simulink model "second_task"  (R2023a)
settings: Solver=VariableStepAuto  StartTime=0.0  StopTime=Tdes  RelTol=1e-3
undefined symbols (not defined in the file): axang2rotm, j, k1e1, k1e2, k2e1, k2e2, kr, ks, kw, n, nd, q0, vs_des
settings Model: Creator=Nabil Samaan  LastModifiedBy=dvogureckiy99
settings DebuggingCC: UnconnectedInputMsg=warning  UnconnectedOutputMsg=warning  UnconnectedLineMsg=warning
settings ModelReferenceCC: EnableRefExpFcnMdlSchedulingChecks=on
settings RTWCC: DLArmComputeVersion=19.05

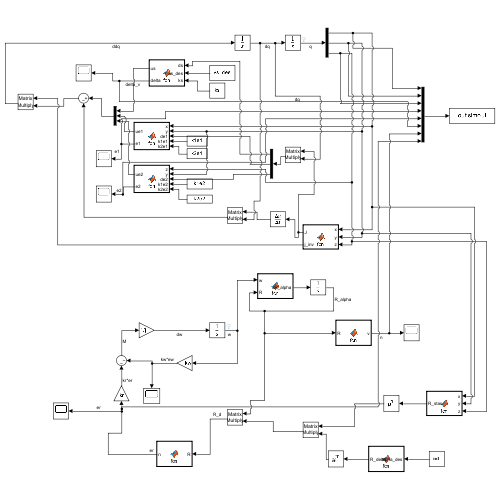
[thumbnail: Simulink's stored preview of the top-level diagram]
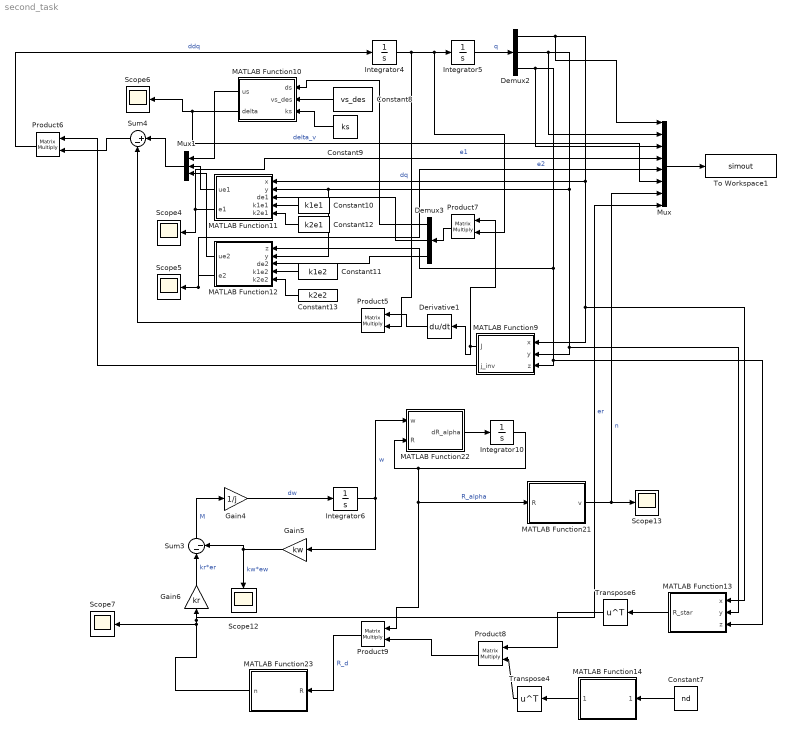
== system second_task ==
  Constant10 : Constant  Value=k1e1
  Constant11 : Constant  Value=k1e2
  Constant12 : Constant  Value=k2e1
  Constant13 : Constant  Value=k2e2
  Constant7 : Constant  Value=nd
  Constant8 : Constant  Value=vs_des
  Constant9 : Constant  Value=ks
  Demux2 : Demux  Outputs=3
  Demux3 : Demux  Outputs=3
  Derivative1 : Derivative  CoefficientInTFapproximation=0.001
  Gain4 : Gain  Gain=1/j
  Gain5 : Gain  Gain=kw
  Gain6 : Gain  Gain=kr
  Integrator10 : Integrator  InitialCondition=axang2rotm([n / norm(n) , norm(n)]);
  Integrator4 : Integrator
  Integrator5 : Integrator  InitialCondition=q0
  Integrator6 : Integrator  InitialCondition=[0;0;0]
  MATLAB Function10 : MATLAB Function  TreatAsAtomicUnit=on
  MATLAB Function11 : MATLAB Function  TreatAsAtomicUnit=on
  MATLAB Function12 : MATLAB Function  TreatAsAtomicUnit=on
  MATLAB Function13 : MATLAB Function  TreatAsAtomicUnit=on
  MATLAB Function14 : MATLAB Function  TreatAsAtomicUnit=on
  MATLAB Function21 : MATLAB Function  TreatAsAtomicUnit=on
  MATLAB Function22 : MATLAB Function  TreatAsAtomicUnit=on
  MATLAB Function23 : MATLAB Function  TreatAsAtomicUnit=on
  MATLAB Function9 : MATLAB Function  TreatAsAtomicUnit=on
  Mux : Mux  Inputs=8
  Mux1 : Mux  Inputs=3
  Product{5..9} (5 alike) : Product  Multiplication=Matrix(*)
  Scope{4..7,12..13} (6 alike) : Scope
  Sum3 : Sum  Inputs=|--
  Sum4 : Sum  Inputs=|+-
  To Workspace1 : ToWorkspace  VariableName=simout  SampleTime=-1
      settings: Save2DSignal=2-D array (concatenate along first dimension)
  Transpose4 : Math  Operator=transpose
  Transpose6 : Math  Operator=transpose
  wires:
  Demux3/1 -> MATLAB Function10/1(ds)
  Constant10/1 -> MATLAB Function11/4(k1e1)
  Gain6/1 -> Sum3/1  "kr*er"
  Product7/1 -> Demux3/1
  MATLAB Function12/2(e2) -> Mux/5, Scope5/1  "e2"
  MATLAB Function14/1(R_delta) -> Transpose4/1
  Gain4/1 -> Integrator6/1  "dw"
  Integrator6/1 -> MATLAB Function22/1(w), Gain5/1  "w"
  Sum3/1 -> Gain4/1  "M"
  MATLAB Function10/2(delta) -> Mux/6, Scope6/1  "delta_v"
  Constant12/1 -> MATLAB Function11/5(k2e1)
  MATLAB Function11/2(e1) -> Scope4/1, Mux/4  "e1"
  Constant13/1 -> MATLAB Function12/5(k2e2)
  MATLAB Function11/1(ue1) -> Mux1/2
  Constant11/1 -> MATLAB Function12/4(k1e2)
  Constant7/1 -> MATLAB Function14/1(alpha_des)
  Gain5/1 -> Scope12/1, Sum3/2  "kw*ew"
  Product6/1 -> Integrator4/1  "ddq"
  Constant9/1 -> MATLAB Function10/3(ks)
  MATLAB Function12/1(ue2) -> Mux1/3
  MATLAB Function9/2(j_inv) -> Product6/1
  Constant8/1 -> MATLAB Function10/2(vs_des)
  Mux1/1 -> Sum4/1
  Demux3/2 -> MATLAB Function11/3(de1)
  Product9/1 -> MATLAB Function23/1(R)  "R_d"
  Derivative1/1 -> Product5/1
  Demux3/3 -> MATLAB Function12/3(de2)
  Product5/1 -> Sum4/2
  MATLAB Function10/1(us) -> Mux1/1
  MATLAB Function9/1(J) -> Derivative1/1, Product7/1
  Integrator5/1 -> Demux2/1  "q"
  Sum4/1 -> Product6/2
  Integrator4/1 -> Product5/2, Product7/2, Integrator5/1  "dq"
  Integrator10/1 -> MATLAB Function22/2(R), MATLAB Function21/1(R), Product9/1  "R_alpha"
  MATLAB Function22/1(dR_alpha) -> Integrator10/1
  MATLAB Function21/1(v) -> Mux/7, Scope13/1  "n"
  Demux2/1 -> Mux/1, MATLAB Function11/1(x), MATLAB Function13/1(x), MATLAB Function9/1(x)
  Demux2/2 -> Mux/2, MATLAB Function9/2(y), MATLAB Function13/2(y), MATLAB Function12/2(y), MATLAB Function11/2(y)
  Demux2/3 -> Mux/3, MATLAB Function12/1(z), MATLAB Function13/3(z), MATLAB Function9/3(z)
  Transpose4/1 -> Product8/2
  MATLAB Function13/1(R_star) -> Transpose6/1
  Transpose6/1 -> Product8/1
  MATLAB Function23/1(n) -> Mux/8, Gain6/1, Scope7/1  "er"
  Product8/1 -> Product9/2
  Mux/1 -> To Workspace1/1

== matlab function second_task/MATLAB Function10 ==
  data: ds input; us output; vs_des input; ks input; delta output
function [us,delta] = fcn(ds,vs_des,ks)

delta=vs_des-ds;

us=ks*delta;

== matlab function second_task/MATLAB Function11 ==
  data: x input; ue1 output; y input; de1 input; k1e1 input; k2e1 input; e1 output
function [ue1,e1] = fcn(x,y,de1,k1e1,k2e1)

e1= 0.4*x^2 + 0.8*y^2 -225;
ue1=-k1e1*de1-k2e1*e1;

== matlab function second_task/MATLAB Function12 ==
  data: z input; ue2 output; y input; de2 input; k1e2 input; k2e2 input; e2 output
function [ue2,e2] = fcn(z,y,de2,k1e2,k2e2)

e2= z+0.25*y^2-3;
ue2=-k1e2*de2-k2e2*e2;

== matlab function second_task/MATLAB Function13 ==
  data: x input; R_star output; y input; z input
function R_star= fcn(x,y,z)

gf1=[0.8*x;1.6*y;0];
gf2=[0;0.5*y;1];
c=cross(gf1,gf2);
j1=c/norm(c);
j2=gf1/norm(gf1);
cc=cross(c,gf1);
j3=cc/norm(cc);

R_star=[j1';j2';j3'];

== matlab function second_task/MATLAB Function14 ==
  data: alpha_des input; R_delta output
function R_delta = fcn(alpha_des)


R_delta= axang2rotm([alpha_des' / norm(alpha_des) , norm(alpha_des)]);

== matlab function second_task/MATLAB Function9 ==
  data: x input; J output; y input; z input; j_inv output
function [J ,j_inv]= fcn(x,y,z)

gf1=[0.8*x;1.6*y;0];
gf2=[0;0.5*y;1];
c=cross(gf1,gf2);
j1=c/norm(c);
j2=gf1/norm(gf1);
j3=gf2/norm(gf2);

J=[j1';j2';j3'];
j_inv=J^(-1);

== matlab function second_task/MATLAB Function21 ==
  data: v output; R input
function v= fcn(R)


p = rotm2axang(R);
v = p(1:3)*p(4);

== matlab function second_task/MATLAB Function22 ==
  data: w input; dR_alpha output; R input
function dR_alpha= fcn(w,R)


s=[0 w(3) -w(2);-w(3) 0 w(1);w(2) -w(1) 0];

dR_alpha=s*R;

== matlab function second_task/MATLAB Function23 ==
  data: R input; n output
function n= fcn(R)

r= R-R';

p = rotm2axang(r);

v = p(1:3)*p(4);

n=0.5*v;
